simulink model "nar_test"  (Simulink 7.8)
settings: Solver=ode45  StartTime=0.0  StopTime=5000  RelTol=1e-3
undefined symbols (not defined in the file or in its folder): pfb_coeff_gen_calc
libraries: xbsIndex_r4 x1069, casper_library_misc x63, xps_library x35, casper_library_delays x19, xbsReplacements_r4 x10, gavrt_library x4, simulink x1
(part 3 of 14)

== system nar_test/pipeline1 ==
  d : Inport
  Register0 : xbsIndex_r4/Register  init=0  rst=off  en=off  dbl_ovrd=off  block_type=register
      settings: block_version=11.4
  q : Outport
  wires:
  d/1 -> Register0/1
  Register0/1 -> q/1

== system nar_test/pipeline10 ==
  d : Inport
  Register0 : xbsIndex_r4/Register  init=0  rst=off  en=off  dbl_ovrd=off  block_type=register
      settings: block_version=11.4
  q : Outport
  wires:
  d/1 -> Register0/1
  Register0/1 -> q/1

== system nar_test/pipeline11 ==
  d : Inport
  Register0 : xbsIndex_r4/Register  init=0  rst=off  en=off  dbl_ovrd=off  block_type=register
      settings: block_version=11.4
  q : Outport
  wires:
  d/1 -> Register0/1
  Register0/1 -> q/1

== system nar_test/pipeline2 ==
  d : Inport
  Register0 : xbsIndex_r4/Register  init=0  rst=off  en=off  dbl_ovrd=off  block_type=register
      settings: block_version=11.4
  q : Outport
  wires:
  d/1 -> Register0/1
  Register0/1 -> q/1

== system nar_test/pipeline24 ==
  d : Inport
  Register0 : xbsIndex_r4/Register  init=0  rst=off  en=off  dbl_ovrd=off  block_type=register
      settings: block_version=11.4
  q : Outport
  wires:
  d/1 -> Register0/1
  Register0/1 -> q/1

== system nar_test/pipeline3 ==
  d : Inport
  Register0 : xbsIndex_r4/Register  init=0  rst=off  en=off  dbl_ovrd=off  block_type=register
      settings: block_version=11.4
  q : Outport
  wires:
  d/1 -> Register0/1
  Register0/1 -> q/1

== system nar_test/pipeline47 ==
  d : Inport
  Register0 : xbsIndex_r4/Register  init=0  rst=off  en=off  dbl_ovrd=off  block_type=register
      settings: block_version=11.4
  q : Outport
  wires:
  d/1 -> Register0/1
  Register0/1 -> q/1

== system nar_test/pipeline48 ==
  d : Inport
  Register0 : xbsIndex_r4/Register  init=0  rst=off  en=off  dbl_ovrd=off  block_type=register
      settings: block_version=11.4
  q : Outport
  wires:
  d/1 -> Register0/1
  Register0/1 -> q/1

== system nar_test/pipeline51 ==
  d : Inport
  Register0 : xbsIndex_r4/Register  init=0  rst=off  en=off  dbl_ovrd=off  block_type=register
      settings: block_version=11.4
  q : Outport
  wires:
  d/1 -> Register0/1
  Register0/1 -> q/1

== system nar_test/pl ==
  In1 : Inport
  In2 : Inport  Port=2
  In3 : Inport  Port=3
  In4 : Inport  Port=4
  In5 : Inport  Port=5
  In6 : Inport  Port=6
  In7 : Inport  Port=7
  In8 : Inport  Port=8
  pipeline10 : Subsystem  AncestorBlock=casper_library_delays/pipeline  mask(pipeline){latency=1}
      mask help:
      | An explicitly laid-out delay line to avoid mapping to SRL16s
      | for use in pipelining to help achieve timing closure.
      mask init:
      | pipeline_init(gcb,'latency',latency);
      settings: AttributesFormatString=Latency = %<latency>
      mask Display:
      | port_label('input', 1, 'd');
      | port_label('output', 1, 'q');
      | disp(['Z^-', num2str(latency)]);
  pipeline11 : Subsystem  AncestorBlock=casper_library_delays/pipeline  mask(pipeline){latency=1}
      mask help:
      | An explicitly laid-out delay line to avoid mapping to SRL16s
      | for use in pipelining to help achieve timing closure.
      mask init:
      | pipeline_init(gcb,'latency',latency);
      settings: AttributesFormatString=Latency = %<latency>
      mask Display:
      | port_label('input', 1, 'd');
      | port_label('output', 1, 'q');
      | disp(['Z^-', num2str(latency)]);
  pipeline12 : Subsystem  AncestorBlock=casper_library_delays/pipeline  mask(pipeline){latency=1}
      mask help:
      | An explicitly laid-out delay line to avoid mapping to SRL16s
      | for use in pipelining to help achieve timing closure.
      mask init:
      | pipeline_init(gcb,'latency',latency);
      settings: AttributesFormatString=Latency = %<latency>
      mask Display:
      | port_label('input', 1, 'd');
      | port_label('output', 1, 'q');
      | disp(['Z^-', num2str(latency)]);
  pipeline13 : Subsystem  AncestorBlock=casper_library_delays/pipeline  mask(pipeline){latency=1}
      mask help:
      | An explicitly laid-out delay line to avoid mapping to SRL16s
      | for use in pipelining to help achieve timing closure.
      mask init:
      | pipeline_init(gcb,'latency',latency);
      settings: AttributesFormatString=Latency = %<latency>
      mask Display:
      | port_label('input', 1, 'd');
      | port_label('output', 1, 'q');
      | disp(['Z^-', num2str(latency)]);
  pipeline14 : Subsystem  AncestorBlock=casper_library_delays/pipeline  mask(pipeline){latency=1}
      mask help:
      | An explicitly laid-out delay line to avoid mapping to SRL16s
      | for use in pipelining to help achieve timing closure.
      mask init:
      | pipeline_init(gcb,'latency',latency);
      settings: AttributesFormatString=Latency = %<latency>
      mask Display:
      | port_label('input', 1, 'd');
      | port_label('output', 1, 'q');
      | disp(['Z^-', num2str(latency)]);
  pipeline15 : Subsystem  AncestorBlock=casper_library_delays/pipeline  mask(pipeline){latency=1}
      mask help:
      | An explicitly laid-out delay line to avoid mapping to SRL16s
      | for use in pipelining to help achieve timing closure.
      mask init:
      | pipeline_init(gcb,'latency',latency);
      settings: AttributesFormatString=Latency = %<latency>
      mask Display:
      | port_label('input', 1, 'd');
      | port_label('output', 1, 'q');
      | disp(['Z^-', num2str(latency)]);
  pipeline16 : Subsystem  AncestorBlock=casper_library_delays/pipeline  mask(pipeline){latency=1}
      mask help:
      | An explicitly laid-out delay line to avoid mapping to SRL16s
      | for use in pipelining to help achieve timing closure.
      mask init:
      | pipeline_init(gcb,'latency',latency);
      settings: AttributesFormatString=Latency = %<latency>
      mask Display:
      | port_label('input', 1, 'd');
      | port_label('output', 1, 'q');
      | disp(['Z^-', num2str(latency)]);
  pipeline17 : Subsystem  AncestorBlock=casper_library_delays/pipeline  mask(pipeline){latency=1}
      mask help:
      | An explicitly laid-out delay line to avoid mapping to SRL16s
      | for use in pipelining to help achieve timing closure.
      mask init:
      | pipeline_init(gcb,'latency',latency);
      settings: AttributesFormatString=Latency = %<latency>
      mask Display:
      | port_label('input', 1, 'd');
      | port_label('output', 1, 'q');
      | disp(['Z^-', num2str(latency)]);
  Out1 : Outport
  Out2 : Outport  Port=2
  Out3 : Outport  Port=3
  Out4 : Outport  Port=4
  Out5 : Outport  Port=5
  Out6 : Outport  Port=6
  Out7 : Outport  Port=7
  Out8 : Outport  Port=8
  wires:
  In1/1 -> pipeline13/1(d)
  pipeline13/1(q) -> Out1/1
  In2/1 -> pipeline11/1(d)
  pipeline11/1(q) -> Out2/1
  In3/1 -> pipeline10/1(d)
  pipeline10/1(q) -> Out3/1
  In4/1 -> pipeline12/1(d)
  pipeline12/1(q) -> Out4/1
  In5/1 -> pipeline17/1(d)
  pipeline17/1(q) -> Out5/1
  In6/1 -> pipeline15/1(d)
  pipeline15/1(q) -> Out6/1
  In7/1 -> pipeline14/1(d)
  pipeline14/1(q) -> Out7/1
  In8/1 -> pipeline16/1(d)
  pipeline16/1(q) -> Out8/1

== system nar_test/snap_sq_trig_16k_adc ==
  din : Inport
  trig : Inport  Port=2
  we : Inport  Port=3
  Constant : xbsIndex_r4/Constant  const=1  gui_display_data_type=Fixed-point  arith_type=Boolean  n_bits=1  bin_pt=0  preci_type=Single  exp_width=8  frac_width=24  explicit_period=on  period=1  equ=P=C  opselect=C  inp2=PCIN>>17  opr=+  inp1=P  carry=CIN  dbl_ovrd=off  block_type=constant
      settings: block_version=10.1.1
  Constant1 : xbsIndex_r4/Constant  const=1  gui_display_data_type=Fixed-point  arith_type=Boolean  n_bits=1  bin_pt=0  preci_type=Single  exp_width=8  frac_width=24  explicit_period=on  period=1  equ=P=C  opselect=C  inp2=PCIN>>17  opr=+  inp1=P  carry=CIN  dbl_ovrd=off  block_type=constant
      settings: block_version=10.1.1
  Constant13 : Constant
  Constant2 : xbsIndex_r4/Constant  const=1  gui_display_data_type=Fixed-point  arith_type=Boolean  n_bits=1  bin_pt=0  preci_type=Single  exp_width=8  frac_width=24  explicit_period=on  period=1  equ=P=C  opselect=C  inp2=PCIN>>17  opr=+  inp1=P  carry=CIN  dbl_ovrd=off  block_type=constant
      settings: block_version=10.1.1
  Inverter : xbsIndex_r4/Inverter  en=off  latency=0  dbl_ovrd=off  block_type=inv
      settings: xl_area=[0, 0, 0, 0, 0, 0, 0]  block_version=10.1.1
  Logical1 : xbsIndex_r4/Logical  logical_function=AND  inputs=2  en=off  latency=0  precision=Full  arith_type=Unsigned  n_bits=8  bin_pt=2  align_bp=on  dbl_ovrd=off  block_type=logical
      settings: xl_area=[0, 0, 0, 0, 0, 0, 0]  block_version=10.1.1
  Mux1 : xbsIndex_r4/Mux  inputs=2  en=off  latency=0  precision=Full  arith_type="Signed  (2's comp)"  n_bits=8  bin_pt=2  quantization=Truncate  overflow=Wrap  dbl_ovrd=off  block_type=mux
      settings: xl_area=[0, 0, 0, 0, 0, 0, 0]  block_version=10.1.1
  Mux2 : xbsIndex_r4/Mux  inputs=2  en=off  latency=0  precision=Full  arith_type="Signed  (2's comp)"  n_bits=8  bin_pt=2  quantization=Truncate  overflow=Wrap  dbl_ovrd=off  block_type=mux
      settings: xl_area=[0, 0, 0, 0, 0, 0, 0]  block_version=10.1.1
  Register : xbsIndex_r4/Register  init=0  rst=on  en=on  dbl_ovrd=off  block_type=register
      settings: xl_area=[0, 0, 0, 0, 0, 0, 0]  block_version=10.1.1
  Register1 : xbsIndex_r4/Register  init=0  rst=on  en=on  dbl_ovrd=off  block_type=register
      settings: xl_area=[0, 0, 0, 0, 0, 0, 0]  block_version=10.1.1
  Reinterpret : xbsIndex_r4/Reinterpret  force_arith_type=on  arith_type=Unsigned  force_bin_pt=on  bin_pt=0  block_type=reinterpret
      settings: infoedit="Changes signal type without altering the binary representation.   You can changed the signal between signed and unsigned, and relocate the binary point.<P><P>Hardware notes: In hardware this block costs nothing.<P><P>Example:  Suppose the input is 6 bits wide, signed, with 2 fractional bits, and the output is forced to unsigned with 0 fractional bits.  Then an input of -2.0 (1110.00 in binary 2's complement) becomes an output of 56 (111000 in binary)."  block_version=10.1.1
  addr : xps_library/software register  Tag=xps:sw_reg  io_dir=To Processor  arith_type=Unsigned  bitwidth=32  bin_pt=0  sample_period=1  gw_name=noise_diode13_bb_11x_snap_sq_trig_16k_adc_addr_user_data_in
  bram : Subsystem  Tag=xps:bram  AncestorBlock=xps_library/Shared BRAM  mask{arith_type=Unsigned, addr_width=nsamples, data_width=32, data_bin_pt=0, init_vals=0, sample_rate=1}
      mask prompts: arith_type "Output Data Type"; addr_width "Address width"; data_width "Data Width"; data_bin_pt "Data Binary Point"; init_vals "Initial 32-bit values (simulation only)"; sample_rate "Sample rate"
      mask init:
      | shared_bram_mask;
      mask StyleString: popup(Unsigned|Signed  (2's comp)),edit,popup(8|16|32|64|128),edit,edit,edit
  ctrl : xps_library/software register  Tag=xps:sw_reg  io_dir=From Processor  arith_type=Unsigned  bitwidth=32  bin_pt=0  sample_period=1  gw_name=noise_diode13_bb_11x_snap_sq_trig_16k_adc_ctrl_user_data_out
  enable : xbsIndex_r4/Slice  nbits=1  boolean_output=on  mode=Lower Bit Location + Width  bit1=0  base1=LSB of Input  bit0=0  base0=LSB of Input  dbl_ovrd=off  block_type=slice
      settings: infoedit="Extracts a given range of bits from each input sample and presents it at the output.  The output type is ordinarily unsigned with binary point at zero, but can be Boolean when the slice is one bit wide.<P><P>Hardware notes: In hardware this block costs nothing."  block_version=10.1.1
  freeze_cntr : casper_library_misc/freeze_cntr  CounterBits=nsamples
  posedge : casper_library_misc/posedge  Tag=Rising Edge Detector
  trig1 : xbsIndex_r4/Slice  nbits=1  boolean_output=on  mode=Lower Bit Location + Width  bit1=0  base1=LSB of Input  bit0=1  base0=LSB of Input  dbl_ovrd=off  block_type=slice
      settings: infoedit="Extracts a given range of bits from each input sample and presents it at the output.  The output type is ordinarily unsigned with binary point at zero, but can be Boolean when the slice is one bit wide.<P><P>Hardware notes: In hardware this block costs nothing."  block_version=10.1.1
  valid : xbsIndex_r4/Slice  nbits=1  boolean_output=on  mode=Lower Bit Location + Width  bit1=0  base1=LSB of Input  bit0=2  base0=LSB of Input  dbl_ovrd=off  block_type=slice
      settings: infoedit="Extracts a given range of bits from each input sample and presents it at the output.  The output type is ordinarily unsigned with binary point at zero, but can be Boolean when the slice is one bit wide.<P><P>Hardware notes: In hardware this block costs nothing."  block_version=10.1.1
  wires:
  trig/1 -> Mux2/2
  freeze_cntr/1 -> Register1/1, bram/1(addr)
  enable/1 -> posedge/1
  Register/1 -> freeze_cntr/2
  freeze_cntr/2 -> bram/3(we), Register1/3
  Constant13/1 -> ctrl/1
  Reinterpret/1 -> bram/2(data_in)
  din/1 -> Reinterpret/1
  ctrl/1 -> enable/1, valid/1, trig1/1
  posedge/1 -> Register/3, Register1/2, Inverter/1
  Constant/1 -> Register/1
  Constant1/1 -> Mux2/3
  Mux1/1 -> freeze_cntr/1
  we/1 -> Mux1/2
  Constant2/1 -> Mux1/3
  Register1/1 -> addr/1
  trig1/1 -> Mux2/1
  valid/1 -> Mux1/1
  Logical1/1 -> Register/2
  Inverter/1 -> Logical1/2
  Mux2/1 -> Logical1/1

== system nar_test/snap_sq_trig_adc ==
  din : Inport
  trig : Inport  Port=2
  we : Inport  Port=3
  Constant : xbsIndex_r4/Constant  const=1  gui_display_data_type=Fixed-point  arith_type=Boolean  n_bits=1  bin_pt=0  preci_type=Single  exp_width=8  frac_width=24  explicit_period=on  period=1  equ=P=C  opselect=C  inp2=PCIN>>17  opr=+  inp1=P  carry=CIN  dbl_ovrd=off  block_type=constant
      settings: block_version=10.1.1
  Constant1 : xbsIndex_r4/Constant  const=1  gui_display_data_type=Fixed-point  arith_type=Boolean  n_bits=1  bin_pt=0  preci_type=Single  exp_width=8  frac_width=24  explicit_period=on  period=1  equ=P=C  opselect=C  inp2=PCIN>>17  opr=+  inp1=P  carry=CIN  dbl_ovrd=off  block_type=constant
      settings: block_version=10.1.1
  Constant13 : Constant
  Constant2 : xbsIndex_r4/Constant  const=1  gui_display_data_type=Fixed-point  arith_type=Boolean  n_bits=1  bin_pt=0  preci_type=Single  exp_width=8  frac_width=24  explicit_period=on  period=1  equ=P=C  opselect=C  inp2=PCIN>>17  opr=+  inp1=P  carry=CIN  dbl_ovrd=off  block_type=constant
      settings: block_version=10.1.1
  Inverter : xbsIndex_r4/Inverter  en=off  latency=0  dbl_ovrd=off  block_type=inv
      settings: xl_area=[0, 0, 0, 0, 0, 0, 0]  block_version=10.1.1
  Logical1 : xbsIndex_r4/Logical  logical_function=AND  inputs=2  en=off  latency=0  precision=Full  arith_type=Unsigned  n_bits=8  bin_pt=2  align_bp=on  dbl_ovrd=off  block_type=logical
      settings: xl_area=[0, 0, 0, 0, 0, 0, 0]  block_version=10.1.1
  Mux1 : xbsIndex_r4/Mux  inputs=2  en=off  latency=0  precision=Full  arith_type="Signed  (2's comp)"  n_bits=8  bin_pt=2  quantization=Truncate  overflow=Wrap  dbl_ovrd=off  block_type=mux
      settings: xl_area=[0, 0, 0, 0, 0, 0, 0]  block_version=10.1.1
  Mux2 : xbsIndex_r4/Mux  inputs=2  en=off  latency=0  precision=Full  arith_type="Signed  (2's comp)"  n_bits=8  bin_pt=2  quantization=Truncate  overflow=Wrap  dbl_ovrd=off  block_type=mux
      settings: xl_area=[0, 0, 0, 0, 0, 0, 0]  block_version=10.1.1
  Register : xbsIndex_r4/Register  init=0  rst=on  en=on  dbl_ovrd=off  block_type=register
      settings: xl_area=[0, 0, 0, 0, 0, 0, 0]  block_version=10.1.1
  Register1 : xbsIndex_r4/Register  init=0  rst=on  en=on  dbl_ovrd=off  block_type=register
      settings: xl_area=[0, 0, 0, 0, 0, 0, 0]  block_version=10.1.1
  Reinterpret : xbsIndex_r4/Reinterpret  force_arith_type=on  arith_type=Unsigned  force_bin_pt=on  bin_pt=0  block_type=reinterpret
      settings: infoedit="Changes signal type without altering the binary representation.   You can changed the signal between signed and unsigned, and relocate the binary point.<P><P>Hardware notes: In hardware this block costs nothing.<P><P>Example:  Suppose the input is 6 bits wide, signed, with 2 fractional bits, and the output is forced to unsigned with 0 fractional bits.  Then an input of -2.0 (1110.00 in binary 2's complement) becomes an output of 56 (111000 in binary)."  block_version=10.1.1
  addr : xps_library/software register  Tag=xps:sw_reg  io_dir=To Processor  arith_type=Unsigned  bitwidth=32  bin_pt=0  sample_period=1  gw_name=noise_diode13_bb_11x_snap_sq_trig_adc_addr_user_data_in
  bram : Subsystem  Tag=xps:bram  AncestorBlock=xps_library/Shared BRAM  mask{arith_type=Unsigned, addr_width=nsamples, data_width=32, data_bin_pt=0, init_vals=0, sample_rate=1}
      mask prompts: arith_type "Output Data Type"; addr_width "Address width"; data_width "Data Width"; data_bin_pt "Data Binary Point"; init_vals "Initial 32-bit values (simulation only)"; sample_rate "Sample rate"
      mask init:
      | shared_bram_mask;
      mask StyleString: popup(Unsigned|Signed  (2's comp)),edit,popup(8|16|32|64|128),edit,edit,edit
  ctrl : xps_library/software register  Tag=xps:sw_reg  io_dir=From Processor  arith_type=Unsigned  bitwidth=32  bin_pt=0  sample_period=1  gw_name=noise_diode13_bb_11x_snap_sq_trig_adc_ctrl_user_data_out
  enable : xbsIndex_r4/Slice  nbits=1  boolean_output=on  mode=Lower Bit Location + Width  bit1=0  base1=LSB of Input  bit0=0  base0=LSB of Input  dbl_ovrd=off  block_type=slice
      settings: infoedit="Extracts a given range of bits from each input sample and presents it at the output.  The output type is ordinarily unsigned with binary point at zero, but can be Boolean when the slice is one bit wide.<P><P>Hardware notes: In hardware this block costs nothing."  block_version=10.1.1
  freeze_cntr : casper_library_misc/freeze_cntr  CounterBits=nsamples
  posedge : casper_library_misc/posedge  Tag=Rising Edge Detector
  trig1 : xbsIndex_r4/Slice  nbits=1  boolean_output=on  mode=Lower Bit Location + Width  bit1=0  base1=LSB of Input  bit0=1  base0=LSB of Input  dbl_ovrd=off  block_type=slice
      settings: infoedit="Extracts a given range of bits from each input sample and presents it at the output.  The output type is ordinarily unsigned with binary point at zero, but can be Boolean when the slice is one bit wide.<P><P>Hardware notes: In hardware this block costs nothing."  block_version=10.1.1
  valid : xbsIndex_r4/Slice  nbits=1  boolean_output=on  mode=Lower Bit Location + Width  bit1=0  base1=LSB of Input  bit0=2  base0=LSB of Input  dbl_ovrd=off  block_type=slice
      settings: infoedit="Extracts a given range of bits from each input sample and presents it at the output.  The output type is ordinarily unsigned with binary point at zero, but can be Boolean when the slice is one bit wide.<P><P>Hardware notes: In hardware this block costs nothing."  block_version=10.1.1
  wires:
  Mux2/1 -> Logical1/1
  Inverter/1 -> Logical1/2
  Logical1/1 -> Register/2
  valid/1 -> Mux1/1
  trig1/1 -> Mux2/1
  Register1/1 -> addr/1
  Constant2/1 -> Mux1/3
  we/1 -> Mux1/2
  Mux1/1 -> freeze_cntr/1
  Constant1/1 -> Mux2/3
  Constant/1 -> Register/1
  posedge/1 -> Inverter/1, Register1/2, Register/3
  ctrl/1 -> trig1/1, valid/1, enable/1
  din/1 -> Reinterpret/1
  Reinterpret/1 -> bram/2(data_in)
  Constant13/1 -> ctrl/1
  freeze_cntr/2 -> Register1/3, bram/3(we)
  Register/1 -> freeze_cntr/2
  enable/1 -> posedge/1
  freeze_cntr/1 -> bram/1(addr), Register1/1
  trig/1 -> Mux2/2

== system nar_test/sync ==
  note: Sync pulse
  note: All this system does is create sync pulses. The PPC will see two registers:
      | sync_pps_arm and sync_manual_arm.
      |
      | Setting either of these to high (1) from low (0) will trigger a new sync pulse.
      | This does NOT send a periodic sync pulse.
  rst_in : Inport
  pps_in : Inport  Port=2
  Constant2 : xbsIndex_r4/Constant  const=1  gui_display_data_type=Fixed-point  arith_type=Signed (2's comp)  n_bits=2  bin_pt=0  preci_type=Single  exp_width=8  frac_width=24  explicit_period=on  period=1  equ=P=C  opselect=C  inp2=PCIN>>17  opr=+  inp1=P  carry=CIN  dbl_ovrd=off  block_type=constant
  Constant4 : Constant  Value=0
  Counter : xbsIndex_r4/Counter  cnt_type=Count Limited  cnt_to=1  operation=Up  start_count=0  cnt_by_val=1  arith_type=Unsigned  n_bits=2  bin_pt=0  load_pin=off  rst=off  en=on  explicit_period=on  period=1  dbl_ovrd=off  use_behavioral_HDL=off  implementation=Fabric  block_type=counter
  Delay40 : xbsIndex_r4/Delay  rst=off  infoeditControl=Selection of Reset will increase slice count due to use of real FFs and instead of SRLs  en=off  latency=1  dbl_ovrd=off  reg_retiming=off  block_type=delay
  Relational : xbsIndex_r4/Relational  mode=a<b  en=off  latency=0  dbl_ovrd=off  block_type=relational
  Slice1 : xbsIndex_r4/Slice  nbits=1  boolean_output=on  mode=Lower Bit Location + Width  bit1=0  base1=MSB of Input  bit0=0  base0=LSB of Input  dbl_ovrd=off  block_type=slice
      settings: block_version=10.1.3
  Slice8 : xbsIndex_r4/Slice  nbits=1  boolean_output=on  mode=Lower Bit Location + Width  bit1=0  base1=MSB of Input  bit0=0  base0=LSB of Input  dbl_ovrd=off  block_type=slice
      settings: block_version=10.1.3
  manual_arm : xps_library/software register  Tag=xps:sw_reg  io_dir=From Processor  arith_type=Unsigned  bitwidth=32  bin_pt=0  sample_period=1  gw_name=nar_test_sync_manual_arm_user_data_out
      link override amnesiac_r100_sync_rst_user_data_out: arith_type=Unsigned  n_bits=32  bin_pt=0  period=1
      link override amnesiac_r101_sync_rst_user_data_out: arith_type=Unsigned  n_bits=32  bin_pt=0  period=1
      link override coarse_r01_sync_rst_user_data_out: arith_type=Unsigned  n_bits=32  bin_pt=0  period=1
      link override coarse_r02_sync_rst_user_data_out: arith_type=Unsigned  n_bits=32  bin_pt=0  period=1
      link override coarse_r03_sync_rst_user_data_out: arith_type=Unsigned  n_bits=32  bin_pt=0  period=1
      link override coarse_r04_sync_rst_user_data_out: arith_type=Unsigned  n_bits=32  bin_pt=0  period=1
      link override coarse_r06_sync_rst_user_data_out: arith_type=Unsigned  n_bits=32  bin_pt=0  period=1
      link override coarse_r07_sync_rst_user_data_out: arith_type=Unsigned  n_bits=32  bin_pt=0  period=1
      link override coarse_r08_sync_rst_user_data_out: arith_type=Unsigned  n_bits=32  bin_pt=0  period=1
      link override coarse_r09_sync_rst_user_data_out: arith_type=Unsigned  n_bits=32  bin_pt=0  period=1
      link override coarse_r10_sync_rst_user_data_out: arith_type=Unsigned  n_bits=32  bin_pt=0  period=1
      link override coarse_r12_sync_rst_user_data_out: arith_type=Unsigned  n_bits=32  bin_pt=0  period=1
      link override convert: arith_type=Unsigned  n_bits=32  bin_pt=0
      link override dpad_spec_r101_acc_len_user_data_out: arith_type=Unsigned  n_bits=32  bin_pt=0  period=1
      link override dpad_spec_r102_acc_len_user_data_out: arith_type=Unsigned  n_bits=32  bin_pt=0  period=1
      link override dpad_spec_r103_acc_len_user_data_out: arith_type=Unsigned  n_bits=32  bin_pt=0  period=1
      link override dpad_spec_r104_acc_len_user_data_out: arith_type=Unsigned  n_bits=32  bin_pt=0  period=1
      link override dpad_spec_r105_acc_len_user_data_out: arith_type=Unsigned  n_bits=32  bin_pt=0  period=1
      link override dpad_spec_r106_fft_shift_user_data_out: arith_type=Unsigned  n_bits=32  bin_pt=0  period=1
      link override dpad_spec_r107_fft_shift_user_data_out: arith_type=Unsigned  n_bits=32  bin_pt=0  period=1
      link override dpad_spec_r108_fft_shift_user_data_out: arith_type=Unsigned  n_bits=32  bin_pt=0  period=1
      link override dpad_spec_r109_fft_shift_user_data_out: arith_type=Unsigned  n_bits=32  bin_pt=0  period=1
      link override dpad_spec_r111_fft_shift_user_data_out: arith_type=Unsigned  n_bits=32  bin_pt=0  period=1
      link override qdr_single_r01_sync_rst_user_data_out: arith_type=Unsigned  n_bits=32  bin_pt=0  period=1
      link override qdr_single_r02_sync_rst_user_data_out: arith_type=Unsigned  n_bits=32  bin_pt=0  period=1
      link override qdr_single_r04_sync_rst_user_data_out: arith_type=Unsigned  n_bits=32  bin_pt=0  period=1
      link override r_spec_2048_r102_acc_len_user_data_out: arith_type=Unsigned  n_bits=32  bin_pt=0  period=1
      link override r_spec_2048_r102_nosim_acc_len_user_data_out: arith_type=Unsigned  n_bits=32  bin_pt=0  period=1
      link override r_spec_2048_r103_acc_len_user_data_out: arith_type=Unsigned  n_bits=32  bin_pt=0  period=1
      link override r_spec_2048_r104_acc_len_user_data_out: arith_type=Unsigned  n_bits=32  bin_pt=0  period=1
      link override r_spec_2048_r104_test0_acc_len_user_data_out: arith_type=Unsigned  n_bits=32  bin_pt=0  period=1
      link override r_spec_2048_r104_test_acc_len_user_data_out: arith_type=Unsigned  n_bits=32  bin_pt=0  period=1
      link override r_spec_2048_r105_acc_len_user_data_out: arith_type=Unsigned  n_bits=32  bin_pt=0  period=1
      link override r_spec_test0_acc_len_user_data_out: arith_type=Unsigned  n_bits=32  bin_pt=0  period=1
      link override r_spec_test4_acc_len_user_data_out: arith_type=Unsigned  n_bits=32  bin_pt=0  period=1
      link override roach_spec_acc_len_user_data_out: arith_type=Unsigned  n_bits=32  bin_pt=0  period=1
      link override roach_spec_no10gbe_acc_len_user_data_out: arith_type=Unsigned  n_bits=32  bin_pt=0  period=1
      link override roach_spec_rst_sync_cnt_user_data_out: arith_type=Unsigned  n_bits=32  bin_pt=0  period=1
      link override the_drowned_world_r100_fft_shift_user_data_out: arith_type=Unsigned  n_bits=32  bin_pt=0  period=1
      link override the_drowned_world_r101_fft_shift_user_data_out: arith_type=Unsigned  n_bits=32  bin_pt=0  period=1
      link override the_drowned_world_r102_fft_shift_user_data_out: arith_type=Unsigned  n_bits=32  bin_pt=0  period=1
      link override the_drowned_world_r103_fft_shift_user_data_out: arith_type=Unsigned  n_bits=32  bin_pt=0  period=1
      link override the_drowned_world_r104_fft_shift_user_data_out: arith_type=Unsigned  n_bits=32  bin_pt=0  period=1
      link override the_drowned_world_r105_sync_rst_user_data_out: arith_type=Unsigned  n_bits=32  bin_pt=0  period=1
      link override the_drowned_world_r106_sync_rst_user_data_out: arith_type=Unsigned  n_bits=32  bin_pt=0  period=1
      link override the_drowned_world_r107_sync_rst_user_data_out: arith_type=Unsigned  n_bits=32  bin_pt=0  period=1
      link override the_drowned_world_r108_sync_rst_user_data_out: arith_type=Unsigned  n_bits=32  bin_pt=0  period=1
      link override the_drowned_world_r109_sync_rst_user_data_out: arith_type=Unsigned  n_bits=32  bin_pt=0  period=1
      link override the_drowned_world_r110_sync_rst_user_data_out: arith_type=Unsigned  n_bits=32  bin_pt=0  period=1
      link override toast_256ch_16bit_r02_sync_rst_user_data_out: arith_type=Unsigned  n_bits=32  bin_pt=0  period=1
      link override toast_256ch_16bit_r04_sync_rst_user_data_out: arith_type=Unsigned  n_bits=32  bin_pt=0  period=1
      link override toast_256ch_16bit_r05_sync_rst_user_data_out: arith_type=Unsigned  n_bits=32  bin_pt=0  period=1
  or2 : xbsIndex_r4/Logical  logical_function=OR  inputs=4  en=off  latency=1  precision=Full  arith_type=Unsigned  n_bits=16  bin_pt=0  align_bp=off  dbl_ovrd=off  block_type=logical
  posedge1 : casper_library_misc/posedge  Tag=Rising Edge Detector
  posedge2 : casper_library_misc/posedge  Tag=Rising Edge Detector
  pps : Subsystem
  Out1 : Outport
  wires:
  manual_arm/1 -> Delay40/1
  Delay40/1 -> Slice8/1
  Slice8/1 -> posedge2/1
  pps/1(Out1) -> or2/2
  posedge2/1 -> or2/3
  rst_in/1 -> or2/1
  or2/1 -> Out1/1
  pps_in/1 -> pps/1(In1)
  Constant4/1 -> manual_arm/1
  Slice1/1 -> posedge1/1
  posedge1/1 -> or2/4
  Counter/1 -> Relational/1
  Relational/1 -> Slice1/1, Counter/1
  Constant2/1 -> Relational/2

== system nar_test/nar/bit_fluff1 ==
  In1 : Inport
  In2 : Inport  Port=2
  Convert : xbsIndex_r4/Convert  gui_display_data_type=Fixed-point  arith_type="Signed  (2's comp)"  n_bits=bits_out  bin_pt=bits_out-1  float_type=Single  exp_bits=8  fraction_bits=24  quantization=Truncate  overflow=Wrap  en=off  latency=0  dbl_ovrd=off  pipeline=off  block_type=convert
  Convert1 : xbsIndex_r4/Convert  gui_display_data_type=Fixed-point  arith_type="Signed  (2's comp)"  n_bits=bits_out  bin_pt=bits_out-1  float_type=Single  exp_bits=8  fraction_bits=24  quantization=Truncate  overflow=Wrap  en=off  latency=0  dbl_ovrd=off  pipeline=off  block_type=convert
  Reinterpret : xbsIndex_r4/Reinterpret  force_arith_type=off  arith_type=Unsigned  force_bin_pt=on  bin_pt=bits_in-1  block_type=reinterpret
  Reinterpret1 : xbsIndex_r4/Reinterpret  force_arith_type=off  arith_type=Unsigned  force_bin_pt=on  bin_pt=bits_in-1  block_type=reinterpret
  Out1 : Outport
  Out2 : Outport  Port=2
  wires:
  Reinterpret1/1 -> Convert1/1
  Reinterpret/1 -> Convert/1
  In1/1 -> Reinterpret/1
  Convert/1 -> Out1/1
  In2/1 -> Reinterpret1/1
  Convert1/1 -> Out2/1

== system nar_test/nar/bit_fluff2 ==
  In1 : Inport
  In2 : Inport  Port=2
  Convert : xbsIndex_r4/Convert  gui_display_data_type=Fixed-point  arith_type="Signed  (2's comp)"  n_bits=bits_out  bin_pt=bits_out-1  float_type=Single  exp_bits=8  fraction_bits=24  quantization=Truncate  overflow=Wrap  en=off  latency=0  dbl_ovrd=off  pipeline=off  block_type=convert
  Convert1 : xbsIndex_r4/Convert  gui_display_data_type=Fixed-point  arith_type="Signed  (2's comp)"  n_bits=bits_out  bin_pt=bits_out-1  float_type=Single  exp_bits=8  fraction_bits=24  quantization=Truncate  overflow=Wrap  en=off  latency=0  dbl_ovrd=off  pipeline=off  block_type=convert
  Reinterpret : xbsIndex_r4/Reinterpret  force_arith_type=off  arith_type=Unsigned  force_bin_pt=on  bin_pt=bits_in-1  block_type=reinterpret
  Reinterpret1 : xbsIndex_r4/Reinterpret  force_arith_type=off  arith_type=Unsigned  force_bin_pt=on  bin_pt=bits_in-1  block_type=reinterpret
  Out1 : Outport
  Out2 : Outport  Port=2
  wires:
  Convert1/1 -> Out2/1
  In2/1 -> Reinterpret1/1
  Convert/1 -> Out1/1
  In1/1 -> Reinterpret/1
  Reinterpret/1 -> Convert/1
  Reinterpret1/1 -> Convert1/1

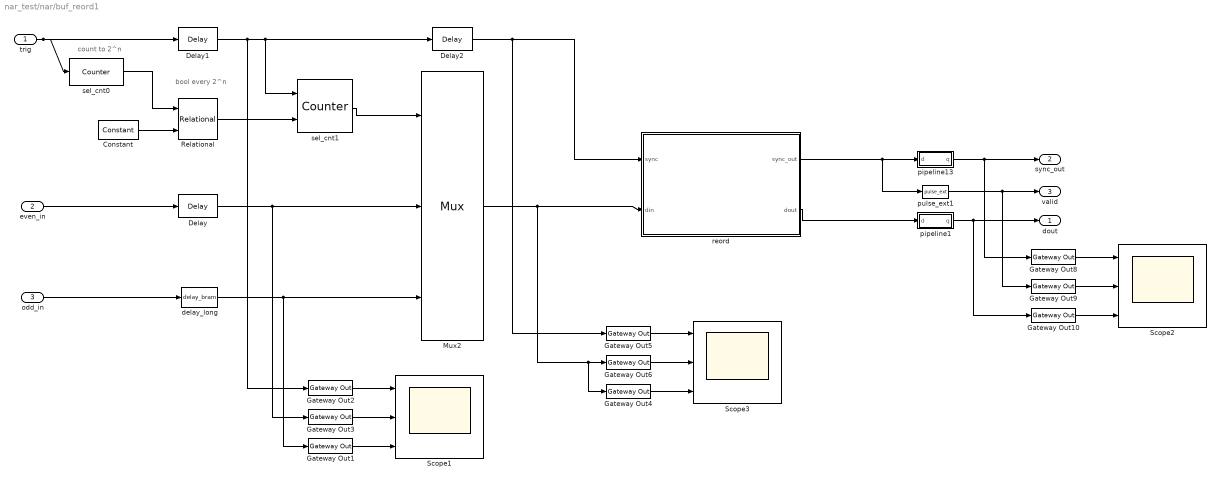
== system nar_test/nar/buf_reord1 ==
  note: count to 2^n
  note: bool every 2^n
  trig : Inport
  even_in : Inport  Port=2
  odd_in : Inport  Port=3
  Constant : xbsIndex_r4/Constant  const=2^(buf_len_bits)-1  gui_display_data_type=Fixed-point  arith_type=Unsigned  n_bits=8  bin_pt=0  preci_type=Single  exp_width=8  frac_width=24  explicit_period=on  period=1  equ=P=C  opselect=C  inp2=PCIN>>17  opr=+  inp1=P  carry=CIN  dbl_ovrd=off  block_type=constant
  Delay : xbsIndex_r4/Delay  rst=off  infoeditControl=Selection of Reset will increase slice count due to use of real FFs and instead of SRLs  en=off  latency=2  dbl_ovrd=off  reg_retiming=off  block_type=delay
  Delay1 : xbsIndex_r4/Delay  rst=off  infoeditControl=Selection of Reset will increase slice count due to use of real FFs and instead of SRLs  en=off  latency=2  dbl_ovrd=off  reg_retiming=off  block_type=delay
  Delay2 : xbsIndex_r4/Delay  rst=off  infoeditControl=Selection of Reset will increase slice count due to use of real FFs and instead of SRLs  en=off  latency=1  dbl_ovrd=off  reg_retiming=off  block_type=delay
  Gateway Out{1..6,8..10} (9 alike) : xbsIndex_r4/Gateway Out  inherit_from_input=off  hdl_port=on  timing_constraint=None  locs_specified=off  LOCs={}  UseAsDAC=off  DACChannel='1'  block_type=gatewayout
      settings: infoedit="Gateway out block.  Converts Xilinx fixed point or floating-point type inputs into ouputs of type Simulink integer, double, or fixed point.<br><br>Hardware notes:  In hardware these blocks become top level output ports or are discarded, depending on how they are configured."
  Mux2 : xbsIndex_r4/Mux  inputs=2  en=off  latency=1  precision=Full  arith_type=Unsigned  n_bits=16  bin_pt=14  quantization=Truncate  overflow=Wrap  dbl_ovrd=off  block_type=mux
  Relational : xbsIndex_r4/Relational  mode=a=b  en=off  latency=2  dbl_ovrd=off  block_type=relational
  Scope1 : Scope  NumInputPorts=3
      settings: YMin=-1~-1~-10000  YMax=1~1~27500
  Scope2 : Scope  NumInputPorts=3
      settings: YMin=-1~-1~-10000  YMax=1~1~27500  SaveName=ScopeData5
  Scope3 : Scope  NumInputPorts=3
      settings: YMin=-1~-1~-10000  YMax=1~1~27500  SaveName=ScopeData3
  delay_long : casper_library_delays/delay_bram  DelayLen=2^(buf_len_bits)+2  bram_latency=4  use_dsp48=on
      link override Counter: use_behavioral_HDL=off  implementation=DSP48  use_rpm=on
  pipeline1 : Subsystem  AncestorBlock=casper_library_delays/pipeline  mask(pipeline){latency=1}
      mask help:
      | An explicitly laid-out delay line to avoid mapping to SRL16s
      | for use in pipelining to help achieve timing closure.
      mask init:
      | pipeline_init(gcb,'latency',latency);
      settings: AttributesFormatString=Latency = %<latency>
      mask Display:
      | port_label('input', 1, 'd');
      | port_label('output', 1, 'q');
      | disp(['Z^-', num2str(latency)]);
  pipeline13 : Subsystem  AncestorBlock=casper_library_delays/pipeline  mask(pipeline){latency=1}
      mask help:
      | An explicitly laid-out delay line to avoid mapping to SRL16s
      | for use in pipelining to help achieve timing closure.
      mask init:
      | pipeline_init(gcb,'latency',latency);
      settings: AttributesFormatString=Latency = %<latency>
      mask Display:
      | port_label('input', 1, 'd');
      | port_label('output', 1, 'q');
      | disp(['Z^-', num2str(latency)]);
  pulse_ext1 : casper_library_misc/pulse_ext  pulse_len=2^(buf_len_bits+1)
  reord : Subsystem  mask{reorder_vec=[0 8 1 9 2 10 3 11 4 12 5 13 6 14 7 15]}
      mask prompts: reorder_vec "Reorder vector"
  sel_cnt0 : xbsIndex_r4/Counter  cnt_type=Free Running  cnt_to=Inf  operation=Up  start_count=0  cnt_by_val=1  arith_type=Unsigned  n_bits=buf_len_bits  bin_pt=0  load_pin=off  rst=on  en=off  explicit_period=on  period=1  dbl_ovrd=off  use_behavioral_HDL=off  implementation=DSP48  block_type=counter
  sel_cnt1 : xbsIndex_r4/Counter  cnt_type=Free Running  cnt_to=Inf  operation=Up  start_count=0  cnt_by_val=1  arith_type=Unsigned  n_bits=1  bin_pt=0  load_pin=off  rst=on  en=on  explicit_period=on  period=1  dbl_ovrd=off  use_behavioral_HDL=off  implementation=Fabric  block_type=counter
  dout : Outport
  sync_out : Outport  Port=2
  valid : Outport  Port=3
  wires:
  pipeline1/1(q) -> Gateway Out10/1, dout/1
  pipeline13/1(q) -> Gateway Out8/1, sync_out/1
  Relational/1 -> sel_cnt1/2
  odd_in/1 -> delay_long/1
  even_in/1 -> Delay/1
  Gateway Out4/1 -> Scope3/3
  Gateway Out6/1 -> Scope3/2
  Gateway Out5/1 -> Scope3/1
  Gateway Out1/1 -> Scope1/3
  Gateway Out3/1 -> Scope1/2
  Gateway Out2/1 -> Scope1/1
  Delay2/1 -> Gateway Out5/1, reord/1(sync)
  Delay1/1 -> sel_cnt1/1, Delay2/1, Gateway Out2/1
  delay_long/1 -> Gateway Out1/1, Mux2/3
  Delay/1 -> Gateway Out3/1, Mux2/2
  sel_cnt1/1 -> Mux2/1
  Mux2/1 -> Gateway Out4/1, Gateway Out6/1, reord/2(din)
  pulse_ext1/1 -> Gateway Out9/1, valid/1
  Gateway Out10/1 -> Scope2/3
  Gateway Out9/1 -> Scope2/2
  Gateway Out8/1 -> Scope2/1
  reord/1(sync_out) -> pipeline13/1(d), pulse_ext1/1
  reord/2(dout) -> pipeline1/1(d)
  trig/1 -> sel_cnt0/1, Delay1/1
  sel_cnt0/1 -> Relational/1
  Constant/1 -> Relational/2

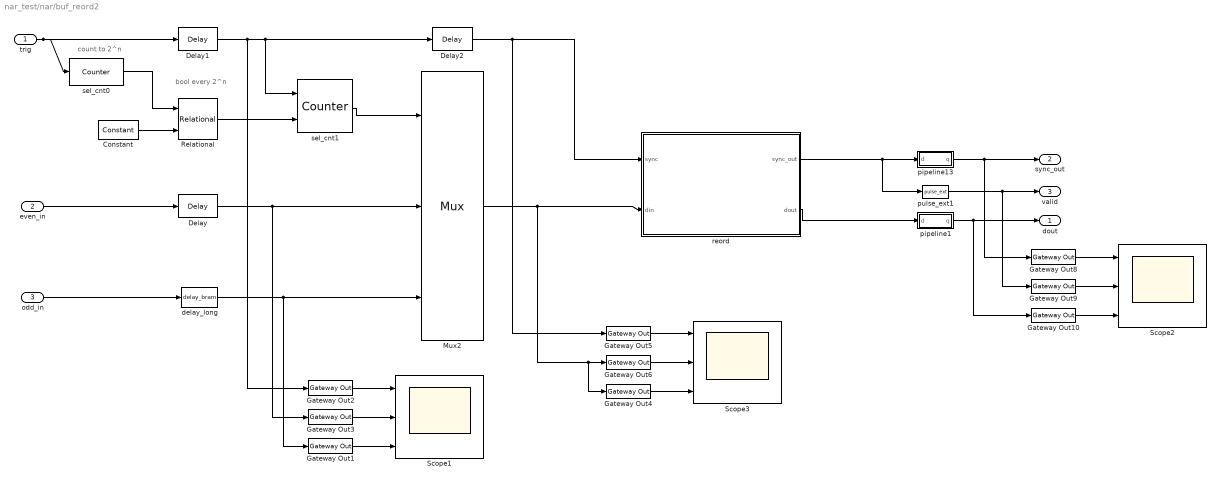
== system nar_test/nar/buf_reord2 ==
  note: bool every 2^n
  note: count to 2^n
  trig : Inport
  even_in : Inport  Port=2
  odd_in : Inport  Port=3
  Constant : xbsIndex_r4/Constant  const=2^(buf_len_bits)-1  gui_display_data_type=Fixed-point  arith_type=Unsigned  n_bits=8  bin_pt=0  preci_type=Single  exp_width=8  frac_width=24  explicit_period=on  period=1  equ=P=C  opselect=C  inp2=PCIN>>17  opr=+  inp1=P  carry=CIN  dbl_ovrd=off  block_type=constant
  Delay : xbsIndex_r4/Delay  rst=off  infoeditControl=Selection of Reset will increase slice count due to use of real FFs and instead of SRLs  en=off  latency=2  dbl_ovrd=off  reg_retiming=off  block_type=delay
  Delay1 : xbsIndex_r4/Delay  rst=off  infoeditControl=Selection of Reset will increase slice count due to use of real FFs and instead of SRLs  en=off  latency=2  dbl_ovrd=off  reg_retiming=off  block_type=delay
  Delay2 : xbsIndex_r4/Delay  rst=off  infoeditControl=Selection of Reset will increase slice count due to use of real FFs and instead of SRLs  en=off  latency=1  dbl_ovrd=off  reg_retiming=off  block_type=delay
  Gateway Out{1..6,8..10} (9 alike) : xbsIndex_r4/Gateway Out  inherit_from_input=off  hdl_port=on  timing_constraint=None  locs_specified=off  LOCs={}  UseAsDAC=off  DACChannel='1'  block_type=gatewayout
      settings: infoedit="Gateway out block.  Converts Xilinx fixed point or floating-point type inputs into ouputs of type Simulink integer, double, or fixed point.<br><br>Hardware notes:  In hardware these blocks become top level output ports or are discarded, depending on how they are configured."
  Mux2 : xbsIndex_r4/Mux  inputs=2  en=off  latency=1  precision=Full  arith_type=Unsigned  n_bits=16  bin_pt=14  quantization=Truncate  overflow=Wrap  dbl_ovrd=off  block_type=mux
  Relational : xbsIndex_r4/Relational  mode=a=b  en=off  latency=2  dbl_ovrd=off  block_type=relational
  Scope1 : Scope  NumInputPorts=3
      settings: YMin=-1~-1~-10000  YMax=1~1~27500
  Scope2 : Scope  NumInputPorts=3
      settings: YMin=-1~-1~-10000  YMax=1~1~27500  SaveName=ScopeData5
  Scope3 : Scope  NumInputPorts=3
      settings: YMin=-1~-1~-10000  YMax=1~1~27500  SaveName=ScopeData3
  delay_long : casper_library_delays/delay_bram  DelayLen=2^(buf_len_bits)+2  bram_latency=4  use_dsp48=on
      link override Counter: use_behavioral_HDL=off  implementation=DSP48  use_rpm=on
  pipeline1 : Subsystem  AncestorBlock=casper_library_delays/pipeline  mask(pipeline){latency=1}
      mask help:
      | An explicitly laid-out delay line to avoid mapping to SRL16s
      | for use in pipelining to help achieve timing closure.
      mask init:
      | pipeline_init(gcb,'latency',latency);
      settings: AttributesFormatString=Latency = %<latency>
      mask Display:
      | port_label('input', 1, 'd');
      | port_label('output', 1, 'q');
      | disp(['Z^-', num2str(latency)]);
  pipeline13 : Subsystem  AncestorBlock=casper_library_delays/pipeline  mask(pipeline){latency=1}
      mask help:
      | An explicitly laid-out delay line to avoid mapping to SRL16s
      | for use in pipelining to help achieve timing closure.
      mask init:
      | pipeline_init(gcb,'latency',latency);
      settings: AttributesFormatString=Latency = %<latency>
      mask Display:
      | port_label('input', 1, 'd');
      | port_label('output', 1, 'q');
      | disp(['Z^-', num2str(latency)]);
  pulse_ext1 : casper_library_misc/pulse_ext  pulse_len=2^(buf_len_bits+1)
  reord : Subsystem  mask{reorder_vec=[0 8 1 9 2 10 3 11 4 12 5 13 6 14 7 15]}
      mask prompts: reorder_vec "Reorder vector"
  sel_cnt0 : xbsIndex_r4/Counter  cnt_type=Free Running  cnt_to=Inf  operation=Up  start_count=0  cnt_by_val=1  arith_type=Unsigned  n_bits=buf_len_bits  bin_pt=0  load_pin=off  rst=on  en=off  explicit_period=on  period=1  dbl_ovrd=off  use_behavioral_HDL=off  implementation=DSP48  block_type=counter
  sel_cnt1 : xbsIndex_r4/Counter  cnt_type=Free Running  cnt_to=Inf  operation=Up  start_count=0  cnt_by_val=1  arith_type=Unsigned  n_bits=1  bin_pt=0  load_pin=off  rst=on  en=on  explicit_period=on  period=1  dbl_ovrd=off  use_behavioral_HDL=off  implementation=Fabric  block_type=counter
  dout : Outport
  sync_out : Outport  Port=2
  valid : Outport  Port=3
  wires:
  Constant/1 -> Relational/2
  sel_cnt0/1 -> Relational/1
  trig/1 -> Delay1/1, sel_cnt0/1
  reord/2(dout) -> pipeline1/1(d)
  reord/1(sync_out) -> pulse_ext1/1, pipeline13/1(d)
  Gateway Out8/1 -> Scope2/1
  Gateway Out9/1 -> Scope2/2
  Gateway Out10/1 -> Scope2/3
  pulse_ext1/1 -> valid/1, Gateway Out9/1
  Mux2/1 -> reord/2(din), Gateway Out6/1, Gateway Out4/1
  sel_cnt1/1 -> Mux2/1
  Delay/1 -> Mux2/2, Gateway Out3/1
  delay_long/1 -> Mux2/3, Gateway Out1/1
  Delay1/1 -> Gateway Out2/1, Delay2/1, sel_cnt1/1
  Delay2/1 -> reord/1(sync), Gateway Out5/1
  Gateway Out2/1 -> Scope1/1
  Gateway Out3/1 -> Scope1/2
  Gateway Out1/1 -> Scope1/3
  Gateway Out5/1 -> Scope3/1
  Gateway Out6/1 -> Scope3/2
  Gateway Out4/1 -> Scope3/3
  even_in/1 -> Delay/1
  odd_in/1 -> delay_long/1
  Relational/1 -> sel_cnt1/2
  pipeline13/1(q) -> sync_out/1, Gateway Out8/1
  pipeline1/1(q) -> dout/1, Gateway Out10/1

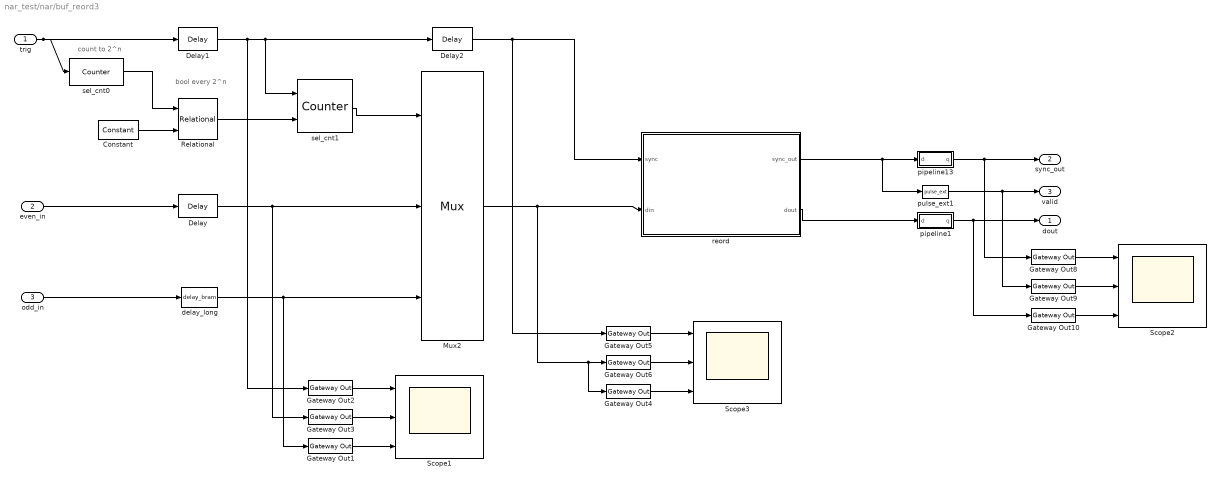
== system nar_test/nar/buf_reord3 ==
  note: count to 2^n
  note: bool every 2^n
  trig : Inport
  even_in : Inport  Port=2
  odd_in : Inport  Port=3
  Constant : xbsIndex_r4/Constant  const=2^(buf_len_bits)-1  gui_display_data_type=Fixed-point  arith_type=Unsigned  n_bits=8  bin_pt=0  preci_type=Single  exp_width=8  frac_width=24  explicit_period=on  period=1  equ=P=C  opselect=C  inp2=PCIN>>17  opr=+  inp1=P  carry=CIN  dbl_ovrd=off  block_type=constant
  Delay : xbsIndex_r4/Delay  rst=off  infoeditControl=Selection of Reset will increase slice count due to use of real FFs and instead of SRLs  en=off  latency=2  dbl_ovrd=off  reg_retiming=off  block_type=delay
  Delay1 : xbsIndex_r4/Delay  rst=off  infoeditControl=Selection of Reset will increase slice count due to use of real FFs and instead of SRLs  en=off  latency=2  dbl_ovrd=off  reg_retiming=off  block_type=delay
  Delay2 : xbsIndex_r4/Delay  rst=off  infoeditControl=Selection of Reset will increase slice count due to use of real FFs and instead of SRLs  en=off  latency=1  dbl_ovrd=off  reg_retiming=off  block_type=delay
  Gateway Out{1..6,8..10} (9 alike) : xbsIndex_r4/Gateway Out  inherit_from_input=off  hdl_port=on  timing_constraint=None  locs_specified=off  LOCs={}  UseAsDAC=off  DACChannel='1'  block_type=gatewayout
      settings: infoedit="Gateway out block.  Converts Xilinx fixed point or floating-point type inputs into ouputs of type Simulink integer, double, or fixed point.<br><br>Hardware notes:  In hardware these blocks become top level output ports or are discarded, depending on how they are configured."
  Mux2 : xbsIndex_r4/Mux  inputs=2  en=off  latency=1  precision=Full  arith_type=Unsigned  n_bits=16  bin_pt=14  quantization=Truncate  overflow=Wrap  dbl_ovrd=off  block_type=mux
  Relational : xbsIndex_r4/Relational  mode=a=b  en=off  latency=2  dbl_ovrd=off  block_type=relational
  Scope1 : Scope  NumInputPorts=3
      settings: YMin=-1~-1~-10000  YMax=1~1~27500
  Scope2 : Scope  NumInputPorts=3
      settings: YMin=-1~-1~-10000  YMax=1~1~27500  SaveName=ScopeData5
  Scope3 : Scope  NumInputPorts=3
      settings: YMin=-1~-1~-10000  YMax=1~1~27500  SaveName=ScopeData3
  delay_long : casper_library_delays/delay_bram  DelayLen=2^(buf_len_bits)+2  bram_latency=4  use_dsp48=on
      link override Counter: use_behavioral_HDL=off  implementation=DSP48  use_rpm=on
  pipeline1 : Subsystem  AncestorBlock=casper_library_delays/pipeline  mask(pipeline){latency=1}
      mask help:
      | An explicitly laid-out delay line to avoid mapping to SRL16s
      | for use in pipelining to help achieve timing closure.
      mask init:
      | pipeline_init(gcb,'latency',latency);
      settings: AttributesFormatString=Latency = %<latency>
      mask Display:
      | port_label('input', 1, 'd');
      | port_label('output', 1, 'q');
      | disp(['Z^-', num2str(latency)]);
  pipeline13 : Subsystem  AncestorBlock=casper_library_delays/pipeline  mask(pipeline){latency=1}
      mask help:
      | An explicitly laid-out delay line to avoid mapping to SRL16s
      | for use in pipelining to help achieve timing closure.
      mask init:
      | pipeline_init(gcb,'latency',latency);
      settings: AttributesFormatString=Latency = %<latency>
      mask Display:
      | port_label('input', 1, 'd');
      | port_label('output', 1, 'q');
      | disp(['Z^-', num2str(latency)]);
  pulse_ext1 : casper_library_misc/pulse_ext  pulse_len=2^(buf_len_bits+1)
  reord : Subsystem  mask{reorder_vec=[0 8 1 9 2 10 3 11 4 12 5 13 6 14 7 15]}
      mask prompts: reorder_vec "Reorder vector"
  sel_cnt0 : xbsIndex_r4/Counter  cnt_type=Free Running  cnt_to=Inf  operation=Up  start_count=0  cnt_by_val=1  arith_type=Unsigned  n_bits=buf_len_bits  bin_pt=0  load_pin=off  rst=on  en=off  explicit_period=on  period=1  dbl_ovrd=off  use_behavioral_HDL=off  implementation=DSP48  block_type=counter
  sel_cnt1 : xbsIndex_r4/Counter  cnt_type=Free Running  cnt_to=Inf  operation=Up  start_count=0  cnt_by_val=1  arith_type=Unsigned  n_bits=1  bin_pt=0  load_pin=off  rst=on  en=on  explicit_period=on  period=1  dbl_ovrd=off  use_behavioral_HDL=off  implementation=Fabric  block_type=counter
  dout : Outport
  sync_out : Outport  Port=2
  valid : Outport  Port=3
  wires:
  pipeline1/1(q) -> Gateway Out10/1, dout/1
  pipeline13/1(q) -> Gateway Out8/1, sync_out/1
  Relational/1 -> sel_cnt1/2
  odd_in/1 -> delay_long/1
  even_in/1 -> Delay/1
  Gateway Out4/1 -> Scope3/3
  Gateway Out6/1 -> Scope3/2
  Gateway Out5/1 -> Scope3/1
  Gateway Out1/1 -> Scope1/3
  Gateway Out3/1 -> Scope1/2
  Gateway Out2/1 -> Scope1/1
  Delay2/1 -> Gateway Out5/1, reord/1(sync)
  Delay1/1 -> sel_cnt1/1, Delay2/1, Gateway Out2/1
  delay_long/1 -> Gateway Out1/1, Mux2/3
  Delay/1 -> Gateway Out3/1, Mux2/2
  sel_cnt1/1 -> Mux2/1
  Mux2/1 -> Gateway Out4/1, Gateway Out6/1, reord/2(din)
  pulse_ext1/1 -> Gateway Out9/1, valid/1
  Gateway Out10/1 -> Scope2/3
  Gateway Out9/1 -> Scope2/2
  Gateway Out8/1 -> Scope2/1
  reord/1(sync_out) -> pipeline13/1(d), pulse_ext1/1
  reord/2(dout) -> pipeline1/1(d)
  trig/1 -> sel_cnt0/1, Delay1/1
  sel_cnt0/1 -> Relational/1
  Constant/1 -> Relational/2
